simulink model "mod3"  (R2019a)
settings: Solver=VariableStepAuto  StartTime=0.0  StopTime=10.0  RelTol=1e-3
libraries: simulink x2
settings Model: Creator=step_oda  LastModifiedBy=bomjz
settings DataIOCC: ReturnWorkspaceOutputs=off
settings DebuggingCC: ArithmeticOperatorsInVariantConditions=warning
settings SFSimCC: SimUseLocalCustomCode=off
settings RTWCC: RTWUseLocalCustomCode=off
settings CodeAppCC: StateflowObjectComments=on

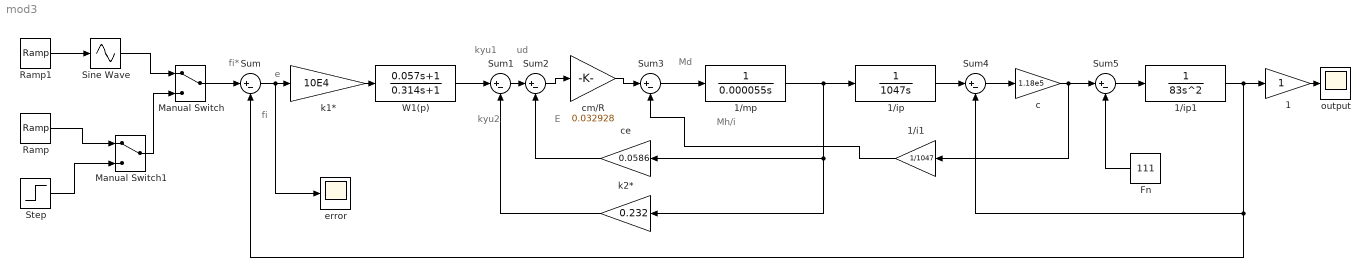
== system mod3 ==
  note: ud
  note: Md
  note: fi
  note: e
  note: fi*
  note: kyu1
  note: kyu2
  note: E
  note: Mh/i
  "1 " : Gain
  1/i1 : Gain  Gain=1/1047
  1/ip : TransferFcn  Denominator=[1047 0]
  1/ip1 : TransferFcn  Denominator=[83 0 0]
  1/mp : TransferFcn  Denominator=[0.000055 0]
  Fn : Constant  Value=111
  Manual Switch : ManualSwitch
  Manual Switch1 : ManualSwitch
  Ramp : simulink/Sources/Ramp  slope=1  start=0  InitialOutput=0
  Ramp1 : simulink/Sources/Ramp  slope=1  start=0  InitialOutput=0
  Sine Wave : Sin  TimeSource=Use external signal  Amplitude=0.09  Frequency=3  SampleTime=0
  Step : Step  Time=0  SampleTime=0
  Sum{,1..5} (6 alike) : Sum  Inputs=|+-
  W1(p) : TransferFcn  Numerator=[0.057 1]  Denominator=[0.314 1]
  c : Gain  Gain=1.18e5
  ce : Gain  Gain=0.0586
  cm/R : Gain  Gain=0.032928
  "error " : Scope
  k1* : Gain  Gain=10E4
  k2* : Gain  Gain=0.232
  output : Scope
  wires:
  Manual Switch/1 -> Sum/1
  Sum/1 -> "error "/1, k1*/1
  k1*/1 -> W1(p)/1
  W1(p)/1 -> Sum1/1
  Sum1/1 -> Sum2/1
  Sum3/1 -> 1/mp/1
  ce/1 -> Sum2/2
  k2*/1 -> Sum1/2
  1/i1/1 -> Sum3/2
  Fn/1 -> Sum5/2
  Sum2/1 -> cm/R/1
  Sine Wave/1 -> Manual Switch/1
  Ramp1/1 -> Sine Wave/1
  Manual Switch1/1 -> Manual Switch/2
  Ramp/1 -> Manual Switch1/1
  Step/1 -> Manual Switch1/2
  cm/R/1 -> Sum3/1
  1/mp/1 -> k2*/1, ce/1, 1/ip/1
  1/ip/1 -> Sum4/1
  Sum4/1 -> c/1
  c/1 -> 1/i1/1, Sum5/1
  Sum5/1 -> 1/ip1/1
  1/ip1/1 -> Sum/2, Sum4/2, "1 "/1
  "1 "/1 -> output/1
